simulink model "Basic_DMT"  (R2014b)
settings: Solver=FixedStepDiscrete  SolverMode=SingleTasking  StartTime=0.0  StopTime=25e-6-14e-9*24  RelTol=1e-3
PreLoadFcn:
  | userName = getenv('UserName');
  | 
  | if strcmp(userName,'Tim')
  | cd C:\Users\Tim\Documents\GitHub\MA_1\Basic_DMT
  | else
  | cd C:\Users\Tim-UML\Documents\GitHub\MA_1\Basic_DMT
  | end
InitFcn:
  | userName = getenv('UserName');
  | 
  | if strcmp(userName,'Tim')
  | cd C:\Users\Tim\Documents\GitHub\MA_1\Basic_DMT
  | else
  | cd C:\Users\Tim-UML\Documents\GitHub\MA_1\Basic_DMT
  | end
values from neighbouring files (symbols this model uses):
  a0 = 0.21194908595403703    (= 0.211949085954)    [initScript.m]
  a1 = 0.576101828091926    (= 0.576101828092)    [initScript.m]
  a2 = a0    (= 0.211949085954)    [initScript.m]
  beta = 1    [initScript.m]
  bitPerSymb = 4    [initScript.m]
  chanDownFact = Tchan/SystemPeriod    [initScript.m]
  fftLen = 16    [initScript.m]
  fftLenActive = fftLenDMT    (= 32)    [initScript.m]
  fftLenDMT = 2*fftLen    (= 32)    [initScript.m]
  GI_Active = GI_LenDMT    (= 0)    [initScript.m]
  GI_Len = 0    [initScript.m]
  GI_LenDMT = 0    [initScript.m]
  M = log2(fftLen)    [initScript.m]
  sysgenSystemPeriod = 4e-9    (= 4e-09)    [initScript.m]
  SystemPeriod = 4e-9    (= 4e-09)    [initScript.m]
  upsampleFactor = 1    [initScript.m]
  usedSubCar = 14    [initScript.m]
undefined symbols (not defined in the file or in its folder): bitCount, get, modu_mode, Tb, Ts
libraries: xbsIndex_r4 x822, commdigbbndam3 x59, simulink x42, dspsigops x7, commrandsrc2 x6, dspbuff3 x4, dspxfrm3 x3, dspswit3 x2, commseqgen2 x1, dsparch4 x1, commutil2 x1, dspsnks4 x1
(part 2 of 10)

== system Basic_DMT/OFDMorDMT ==
  note: 1) Add Subsystem or Model blocks as valid variant choices.
      | 2) You cannot connect blocks at this level. At simulation, connectivity is automatically
      | determined, based on the active variant and port name matching.
  In1 : Inport
  DMT : Subsystem  VariantControl=dmtOfdm==2
  OFDM : Subsystem  VariantControl=dmtOfdm==1
  Out1 : Outport

== system Basic_DMT/PIS  ==
  Sub1 : Inport
  Sub2 : Inport  Port=2
  Sub3 : Inport  Port=3
  Sub4 : Inport  Port=4
  Sub5 : Inport  Port=5
  Sub6 : Inport  Port=6
  Sub7 : Inport  Port=7
  Sub8 : Inport  Port=8
  Sub9 : Inport  Port=9
  Sub10 : Inport  Port=10
  Sub11 : Inport  Port=11
  Sub12 : Inport  Port=12
  Sub13 : Inport  Port=13
  Sub14 : Inport  Port=14
  sg_Bit : Inport  Port=15
  Add3 : Sum  Inputs=+-
  Delay : Delay  DelayLength=1  InitialCondition=0
  Gateway Out : xbsIndex_r4/Gateway Out  inherit_from_input=on  hdl_port=off  rows=1  columns=1  UseAsDAC=off  DACChannel='1'  interface=None  automatic_assignment=on  address_offset=hex2dec('00')  intf_description=''  timing_constraint=None  locs_specified=off  LOCs={}  io_standard={}  block_type=gatewayout
  Mux : Mux  Inputs=14
  Scope5 : Scope  Commented=on  NumInputPorts=3
      settings: YMin=-5~-5~-5  YMax=5~5~5  SaveName=ScopeData29
  Unbuffer : Unbuffer  SampleBasedProcessing=Same as frame based
  Out : Outport
  wires:
  Mux/1 -> Unbuffer/1
  Sub2/1 -> Mux/2
  Sub1/1 -> Mux/1
  Gateway Out/1 -> Scope5/2, Add3/2
  Add3/1 -> Scope5/3
  Unbuffer/1 -> Delay/1
  Delay/1 -> Add3/1, Scope5/1, Out/1
  sg_Bit/1 -> Gateway Out/1
  Sub4/1 -> Mux/4
  Sub3/1 -> Mux/3
  Sub6/1 -> Mux/6
  Sub5/1 -> Mux/5
  Sub8/1 -> Mux/8
  Sub7/1 -> Mux/7
  Sub10/1 -> Mux/10
  Sub9/1 -> Mux/9
  Sub11/1 -> Mux/11
  Sub13/1 -> Mux/13
  Sub14/1 -> Mux/14
  Sub12/1 -> Mux/12

== system Basic_DMT/Receiver ==

== system Basic_DMT/SIP  ==
  S1 : Inport
  Debug1 : Inport  Port=2
  Debug2 : Inport  Port=3
  Add1 : Sum  Inputs=+-
  Assert DIfferent Output : Subsystem
  Buffer : Buffer  N=usedSubCar*bitPerSymb  TreatMby1Signals=One channel
  Constant1 : Constant  Value=0  SampleTime=SystemPeriod
  Data Store Memory : DataStoreMemory  DataStoreName=state  OutDataTypeStr=double
  Data Store Memory1 : DataStoreMemory  DataStoreName=k  OutDataTypeStr=double
  Data Store Memory2 : DataStoreMemory  DataStoreName=loopCount  OutDataTypeStr=double
  Data Store Memory3 : DataStoreMemory  DataStoreName=subCar  InitialValue=1  OutDataTypeStr=double
  Delay : Delay  DelayLength=1  InitialCondition=0
  Delay1 : Delay  DelayLength=65  InitialCondition=0
  Delay2 : Delay  DelayLength=1  InitialCondition=0
  Demux : Demux  Outputs=14
  Index Vector : MultiPortSwitch  DataPortOrder=Zero-based contiguous  Inputs=2  zeroidx=on
  MATLAB Function : MATLAB Function  TreatAsAtomicUnit=on  SystemSampleTime=SystemPeriod
  Queue : dspbuff3/Queue  depth=64  trigger=Non-zero sample  overflow=Dynamic reallocation  pes=Warning  eso=off  fso=off  nso=on  clr=off  clrOutport=off  adf=off
  Scope1 : Scope  NumInputPorts=3
      settings: YMin=0~0~0  YMax=1~1~1  SaveName=ScopeData70
  Scope2 : Scope  NumInputPorts=2
      settings: YMin=0~-0  YMax=1~2  SaveName=ScopeData71
  Scope3 : Scope  NumInputPorts=3
      settings: YMin=0~0~-1  YMax=1~1~1  SaveName=ScopeData73
  Zero-Order Hold : ZeroOrderHold  SampleTime=SystemPeriod
  Zero-Order Hold1 : ZeroOrderHold  SampleTime=Ts
  Sub1 : Outport
  Sub2 : Outport  Port=2
  Sub3 : Outport  Port=3
  Sub4 : Outport  Port=4
  Sub5 : Outport  Port=5
  Sub6 : Outport  Port=6
  Sub7 : Outport  Port=7
  Sub8 : Outport  Port=8
  Sub9 : Outport  Port=9
  Sub10 : Outport  Port=10
  Sub11 : Outport  Port=11
  Sub12 : Outport  Port=12
  Sub13 : Outport  Port=13
  Sub14 : Outport  Port=14
  wires:
  Demux/2 -> Assert DIfferent Output/2(In2), Sub2/1
  Buffer/1 -> Demux/1
  Demux/1 -> Assert DIfferent Output/1(In1), Sub1/1
  Debug1/1 -> Assert DIfferent Output/3(In3)
  Debug2/1 -> Assert DIfferent Output/4(In4)
  Zero-Order Hold/1 -> Zero-Order Hold1/1, Scope2/1, Queue/1
  Demux/3 -> Sub3/1
  Demux/4 -> Sub4/1
  Demux/5 -> Sub5/1
  Demux/6 -> Sub6/1
  Demux/7 -> Sub7/1
  Demux/8 -> Sub8/1
  Demux/9 -> Sub9/1
  Demux/10 -> Sub10/1
  Demux/11 -> Sub11/1
  Demux/14 -> Sub14/1
  Demux/13 -> Sub13/1
  Demux/12 -> Sub12/1
  Queue/1 -> Index Vector/3
  Constant1/1 -> Index Vector/2
  Queue/2 -> Delay/1
  MATLAB Function/1(sel) -> Index Vector/1, Scope1/1
  Delay/1 -> MATLAB Function/1(num), Scope2/2
  Index Vector/1 -> Delay2/1
  Zero-Order Hold1/1 -> Delay1/1
  Add1/1 -> Scope3/3
  Delay1/1 -> Add1/2, Scope3/2
  MATLAB Function/2(push) -> Scope1/2, Queue/2
  MATLAB Function/3(pop) -> Scope1/3, Queue/3
  S1/1 -> Zero-Order Hold/1
  Delay2/1 -> Buffer/1, Scope3/1, Add1/1

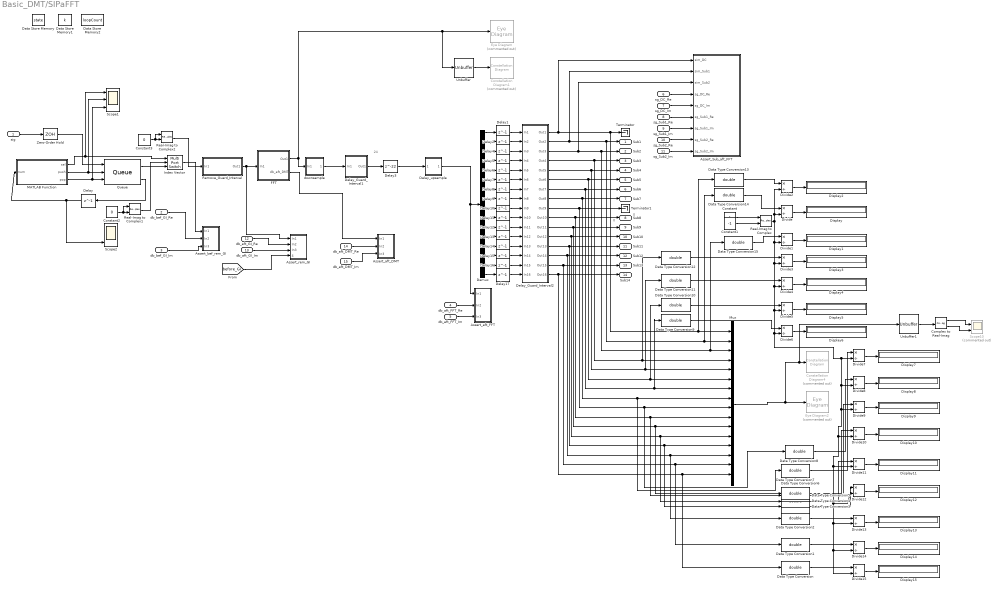
== system Basic_DMT/SIPaFFT ==
  note: 24
  note: 0
  note: 0
  sig : Inport
  db_bef_GI_Re : Inport  Port=2
  db_bef_GI_Im : Inport  Port=3
  db_aft_FFT_Re : Inport  Port=4
  db_aft_FFT_Im : Inport  Port=5
  sg_DC_Re : Inport  Port=6
  sg_DC_Im : Inport  Port=7
  sg_Sub1_Re : Inport  Port=8
  sg_Sub1_Im : Inport  Port=9
  sg_Sub2_Re : Inport  Port=10
  sg_Sub2_Im : Inport  Port=11
  db_aft_GI_Re : Inport  Port=12
  db_aft_GI_Im : Inport  Port=13
  db_aft_DMT_Re : Inport  Port=14
  db_aft_DMT_Im : Inport  Port=15
  Assert_Sub_aft_FFT : Subsystem
  Assert_aft_DMT : Subsystem
  Assert_aft_FFT : Subsystem
  Assert_bef_rem_GI : Subsystem
  Assert_rem_GI : Subsystem
  Complex to Real-Imag : ComplexToRealImag
  Constant : Constant
  Constant1 : Constant  Value=-1
  Constant2 : Constant  Value=0  SampleTime=SystemPeriod
  Constant3 : Constant  Value=0  SampleTime=SystemPeriod
  Constellation Diagram1 : ConstellationDiagram  Commented=on
  Constellation Diagram4 : ConstellationDiagram  Commented=on
  Data Store Memory : DataStoreMemory  DataStoreName=state  OutDataTypeStr=double
  Data Store Memory1 : DataStoreMemory  DataStoreName=k  OutDataTypeStr=double
  Data Store Memory2 : DataStoreMemory  DataStoreName=loopCount  OutDataTypeStr=double
  Data Type Conversion{,1..15} (16 alike) : DataTypeConversion  OutDataTypeStr=double
  Delay : Delay  DelayLength=1  InitialCondition=0
  Delay{1..2,4..17} (16 alike) : Delay  DelayLength=1  InitialCondition=0  InputProcessing=Columns as channels (frame based)
  Delay3 : Delay  DelayLength=22  InitialCondition=0  InputProcessing=Columns as channels (frame based)
  Delay_Guard_Interval1 : Subsystem  Variant=on
  Delay_Guard_Interval2 : Subsystem  Variant=on
  Delay_upsample : Subsystem  Variant=on
  Demux : Demux  Outputs=16
  Display{,1..15} (16 alike) : Display
  Divide{,1..15} (16 alike) : Product  Inputs=*/
  Eye Diagram : EyeDiagram  Commented=on
  Eye Diagram2 : EyeDiagram  Commented=on
  FFT : Subsystem  Variant=on
  Index Vector : MultiPortSwitch  DataPortOrder=Zero-based contiguous  Inputs=2  zeroidx=on
  MATLAB Function : MATLAB Function  TreatAsAtomicUnit=on  SystemSampleTime=SystemPeriod
  Mux : Mux  Inputs=16
  Queue : dspbuff3/Queue  depth=64  trigger=Non-zero sample  overflow=Dynamic reallocation  pes=Warning  eso=off  fso=off  nso=on  clr=off  clrOutport=off  adf=off
  Real-Imag to Complex : RealImagToComplex
  Real-Imag to Complex1 : RealImagToComplex
  Real-Imag to Complex2 : RealImagToComplex
  Remove_Guard_Interval : Subsystem  Variant=on
  Scope1 : Scope  NumInputPorts=3
      settings: YMin=0~0~0  YMax=1~1~1  SaveName=ScopeData75
  Scope10 : Scope  Commented=on  NumInputPorts=2
      settings: YMin=-5~-5  YMax=5~5  SaveName=ScopeData66
  Scope2 : Scope  NumInputPorts=3
      settings: YMin=0~0~0  YMax=1~1~1  SaveName=ScopeData76
  Terminator : Terminator
  Terminator1 : Terminator
  Unbuffer : Unbuffer  SampleBasedProcessing=Same as frame based
  Unbuffer1 : Unbuffer  SampleBasedProcessing=Same as frame based
  Zero-Order Hold : ZeroOrderHold  SampleTime=SystemPeriod
  downsample : Subsystem  Variant=on
  Sub1 : Outport
  Sub2 : Outport  Port=2
  Sub3 : Outport  Port=3
  Sub4 : Outport  Port=4
  Sub5 : Outport  Port=5
  Sub6 : Outport  Port=6
  Sub7 : Outport  Port=7
  Sub8 : Outport  Port=8
  Sub9 : Outport  Port=9
  Sub10 : Outport  Port=10
  Sub11 : Outport  Port=11
  Sub12 : Outport  Port=12
  Sub13 : Outport  Port=13
  Sub14 : Outport  Port=14
  wires:
  Demux/2 -> Delay2/1
  Demux/3 -> Delay4/1
  Demux/1 -> Delay1/1
  Demux/4 -> Delay5/1
  Demux/6 -> Delay7/1
  Demux/5 -> Delay6/1
  Demux/7 -> Delay8/1
  Demux/8 -> Delay9/1
  db_bef_GI_Im/1 -> Assert_bef_rem_GI/3(In3)
  db_bef_GI_Re/1 -> Assert_bef_rem_GI/2(In2)
  db_aft_FFT_Re/1 -> Assert_aft_FFT/2(In2)
  db_aft_FFT_Im/1 -> Assert_aft_FFT/3(In3)
  sg_DC_Re/1 -> Assert_Sub_aft_FFT/4(sg_DC_Re)
  sg_DC_Im/1 -> Assert_Sub_aft_FFT/5(sg_DC_Im)
  sg_Sub1_Re/1 -> Assert_Sub_aft_FFT/6(sg_Sub1_Re)
  sg_Sub1_Im/1 -> Assert_Sub_aft_FFT/7(sg_Sub1_Im)
  sg_Sub2_Re/1 -> Assert_Sub_aft_FFT/8(sg_Sub2_Re)
  sg_Sub2_Im/1 -> Assert_Sub_aft_FFT/9(sg_Sub2_Im)
  Delay3/1 -> Delay_upsample/1(In1)
  Delay1/1 -> Delay_Guard_Interval2/1(In1)
  db_aft_GI_Im/1 -> Assert_rem_GI/3(In3)
  db_aft_GI_Re/1 -> Assert_rem_GI/2(In2)
  [before_GI] -> Assert_rem_GI/4(before_GI)
  Index Vector/1 -> Assert_bef_rem_GI/1(In1)
  Demux/16 -> Delay17/1
  Demux/15 -> Delay16/1
  Demux/14 -> Delay15/1
  Demux/13 -> Delay14/1
  Demux/12 -> Delay13/1
  Demux/11 -> Delay12/1
  Demux/10 -> Delay11/1
  Demux/9 -> Delay10/1
  Delay4/1 -> Delay_Guard_Interval2/3(In3)
  Delay5/1 -> Delay_Guard_Interval2/4(In4)
  Delay2/1 -> Delay_Guard_Interval2/2(In2)
  Delay6/1 -> Delay_Guard_Interval2/5(In5)
  Delay7/1 -> Delay_Guard_Interval2/6(In6)
  Delay8/1 -> Delay_Guard_Interval2/7(In7)
  Delay9/1 -> Delay_Guard_Interval2/8(In8)
  Delay10/1 -> Delay_Guard_Interval2/9(In9)
  Delay11/1 -> Delay_Guard_Interval2/10(In10)
  Delay12/1 -> Delay_Guard_Interval2/11(In11)
  Delay13/1 -> Delay_Guard_Interval2/12(In12)
  Delay14/1 -> Delay_Guard_Interval2/13(In13)
  Delay15/1 -> Delay_Guard_Interval2/14(In14)
  Delay16/1 -> Delay_Guard_Interval2/15(In15)
  Delay17/1 -> Delay_Guard_Interval2/16(In16)
  Delay_Guard_Interval1/1(Out1) -> Delay3/1
  Remove_Guard_Interval/1(Out1) -> FFT/1(In1), Assert_rem_GI/1(In1)
  downsample/1(Out1) -> Delay_Guard_Interval1/1(In1)
  Delay_upsample/1(Out1) -> Assert_aft_FFT/1(In1), Demux/1
  FFT/1(Out1) -> downsample/1(In1), Unbuffer/1, Eye Diagram/1
  db_aft_DMT_Im/1 -> Assert_aft_DMT/3(In3)
  db_aft_DMT_Re/1 -> Assert_aft_DMT/2(In2)
  FFT/2(db_aft_DMT) -> Assert_aft_DMT/1(In1)
  Delay_Guard_Interval2/2(Out2) -> Assert_Sub_aft_FFT/2(sim_Sub1), Data Type Conversion14/1, Mux/2, Sub1/1
  Delay_Guard_Interval2/4(Out4) -> Mux/4, Data Type Conversion12/1, Sub3/1
  Delay_Guard_Interval2/5(Out5) -> Data Type Conversion11/1, Mux/5, Sub4/1
  Delay_Guard_Interval2/6(Out6) -> Data Type Conversion10/1, Mux/6, Sub5/1
  Delay_Guard_Interval2/7(Out7) -> Data Type Conversion9/1, Mux/7, Sub6/1
  Delay_Guard_Interval2/9(Out9) -> Data Type Conversion8/1, Mux/9, Terminator1/1
  Delay_Guard_Interval2/10(Out10) -> Data Type Conversion5/1, Mux/10, Sub8/1
  Delay_Guard_Interval2/12(Out12) -> Data Type Conversion4/1, Mux/12, Sub10/1
  Delay_Guard_Interval2/15(Out15) -> Sub13/1, Data Type Conversion1/1, Mux/15
  Delay_Guard_Interval2/14(Out14) -> Sub12/1, Data Type Conversion2/1, Mux/14
  Delay_Guard_Interval2/13(Out13) -> Sub11/1, Data Type Conversion3/1, Mux/13
  Delay_Guard_Interval2/11(Out11) -> Data Type Conversion6/1, Mux/11, Sub9/1
  Mux/1 -> Unbuffer1/1, Constellation Diagram4/1, Eye Diagram2/1
  Unbuffer/1 -> Constellation Diagram1/1
  Constant/1 -> Real-Imag to Complex/1
  Divide/1 -> Display/1
  Delay_Guard_Interval2/3(Out3) -> Assert_Sub_aft_FFT/3(sim_Sub2), Mux/3, Data Type Conversion15/1, Sub2/1
  Constant1/1 -> Real-Imag to Complex/2
  Divide1/1 -> Display1/1
  Delay_Guard_Interval2/1(Out1) -> Data Type Conversion13/1, Mux/1, Terminator/1, Assert_Sub_aft_FFT/1(sim_DC)
  Real-Imag to Complex/1 -> Divide2/2, Divide/2, Divide15/2, Divide14/2, Divide13/2, Divide12/2, Divide11/2, Divide10/2, Divide9/2, Divide8/2, Divide7/2, Divide6/2, Divide5/2, Divide4/2, Divide3/2, Divide1/2
  Divide2/1 -> Display2/1
  Divide3/1 -> Display3/1
  Divide4/1 -> Display4/1
  Divide5/1 -> Display5/1
  Divide6/1 -> Display6/1
  Divide7/1 -> Display7/1
  Divide8/1 -> Display8/1
  Divide9/1 -> Display9/1
  Divide10/1 -> Display10/1
  Divide11/1 -> Display11/1
  Divide12/1 -> Display12/1
  Divide13/1 -> Display13/1
  Divide14/1 -> Display14/1
  Divide15/1 -> Display15/1
  Delay_Guard_Interval2/16(Out16) -> Data Type Conversion/1, Mux/16, Sub14/1
  Data Type Conversion/1 -> Divide15/1
  Data Type Conversion1/1 -> Divide14/1
  Data Type Conversion2/1 -> Divide13/1
  Data Type Conversion3/1 -> Divide12/1
  Data Type Conversion4/1 -> Divide11/1
  Data Type Conversion5/1 -> Divide9/1
  Data Type Conversion6/1 -> Divide10/1
  Data Type Conversion7/1 -> Divide7/1
  Data Type Conversion8/1 -> Divide8/1
  Data Type Conversion9/1 -> Divide6/1
  Data Type Conversion10/1 -> Divide5/1
  Data Type Conversion11/1 -> Divide4/1
  Data Type Conversion12/1 -> Divide3/1
  Data Type Conversion13/1 -> Divide2/1
  Data Type Conversion14/1 -> Divide/1
  Data Type Conversion15/1 -> Divide1/1
  Unbuffer1/1 -> Complex to Real-Imag/1
  Complex to Real-Imag/1 -> Scope10/1
  Complex to Real-Imag/2 -> Scope10/2
  Delay_Guard_Interval2/8(Out8) -> Data Type Conversion7/1, Mux/8, Sub7/1
  MATLAB Function/3(pop) -> Scope1/3, Queue/3
  MATLAB Function/2(push) -> Scope1/2, Queue/2
  sig/1 -> Zero-Order Hold/1
  Queue/1 -> Index Vector/3
  MATLAB Function/1(sel) -> Scope1/1, Index Vector/1
  Queue/2 -> Delay/1
  Delay/1 -> Scope2/3, MATLAB Function/1(num)
  Constant2/1 -> Real-Imag to Complex1/2, Real-Imag to Complex1/1
  Zero-Order Hold/1 -> Queue/1
  Real-Imag to Complex2/1 -> Remove_Guard_Interval/1(In1)
  Real-Imag to Complex1/1 -> Index Vector/2
  Constant3/1 -> Real-Imag to Complex2/2, Real-Imag to Complex2/1

== system Basic_DMT/Subsystem ==

== system Basic_DMT/Sysgen S//P1 ==
  " System Generator" : xbsIndex_r4/ System Generator  Tag=genX  xilinxfamily=zynq  part=xc7z020  speed=-1  package=clg400  synthesis_tool=Vivado  clock_wrapper=Clock Enables  directory=./netlist  proj_type=Vivado  Synth_file=Vivado Synthesis Defaults  Impl_file=Vivado Implementation Defaults  testbench=on  simulink_period=Ts  sysclk_period=10  dcm_input_clock_period=10  incr_netlist=off  trim_vbits=Everywhere in SubSystem  dbl_ovrd=According to Block Masks  core_generation=According to Block Masks  run_coregen=off  deprecated_control=off  eval_field=0  block_type=sysgen
  Bernoulli Binary Generator : commrandsrc2/Bernoulli Binary Generator  P=0.5  seed=1604198  Ts=Tb  frameBased=off  sampPerFrame=1  orient=off  outDataType=boolean
      settings: AttributesFormatString=|
      | Sample Time= %<Ts>
      | Prob zero=%<P>
  BitBasher : xbsIndex_r4/BitBasher  bitexpr=|  display_expr=on  sr_1=y1  arith_type1=Unsigned  bin_pt1=0  sr_2=y2  arith_type2=Unsigned  bin_pt2=0  sr_3=3  arith_type3=Unsigned  bin_pt3=0  sr_4=4  arith_type4=Unsigned  bin_pt4=0  dbl_ovrd=off  block_type=bitbasher
      | y1={a[7:4]}
      | y2={a[3:0]}
  Buffer : Buffer  N=8  TreatMby1Signals=One channel
  Check Static Range1 : simulink/Model Verification/Check  Static Range  Description=0 <= u <= 0  max=0  max_included=on  min=0  min_included=on  enabled=on  stopWhenAssertionFail=on  export=off  icon=graphic
  Check Static Range2 : simulink/Model Verification/Check  Static Range  Description=0 <= u <= 0  max=0  max_included=on  min=0  min_included=on  enabled=on  stopWhenAssertionFail=on  export=off  icon=graphic
  Clock Probe1 : xbsIndex_r4/Clock Probe  block_type=clkprobe
      settings: infoedit="Clock probe.  Produces an output of type double that mirrors the hardware system clock.<br><br>Hardware notes:  This block is ignored when hardware is generated."
  Counter Limited1 : simulink/Sources/Counter Limited  uplimit=1  tsamp=Tb
  Delay : Delay  DelayLength=1  InitialCondition=0
  Delay1 : Delay  DelayLength=1  InitialCondition=0
  Demux : Demux  Outputs=2
  Gateway In1 : xbsIndex_r4/Gateway In  gui_display_data_type=Fixed-point  arith_type=Unsigned  n_bits=1  bin_pt=0  preci_type=Single  exp_width=8  frac_width=24  rows=1  columns=1  quantization="Round  (unbiased: +/- Inf)"  overflow=Saturate  period=Ts  UseAsADC=off  ADCChannel='1'  interface=None  automatic_assignment=on  address_offset=hex2dec('00')  intf_description=''  timing_constraint=None  locs_specified=off  LOCs={}  io_standard={}  inherit_from_input=off  hdl_port=on  dbl_ovrd=off  block_type=gatewayin
  Gateway Out : xbsIndex_r4/Gateway Out  inherit_from_input=on  hdl_port=off  rows=1  columns=1  UseAsDAC=off  DACChannel='1'  interface=None  automatic_assignment=on  address_offset=hex2dec('00')  intf_description=''  timing_constraint=None  locs_specified=off  LOCs={}  io_standard={}  block_type=gatewayout
  Gateway Out1 : xbsIndex_r4/Gateway Out  inherit_from_input=on  hdl_port=off  rows=1  columns=1  UseAsDAC=off  DACChannel='1'  interface=None  automatic_assignment=on  address_offset=hex2dec('00')  intf_description=''  timing_constraint=None  locs_specified=off  LOCs={}  io_standard={}  block_type=gatewayout
  Manual Switch : ManualSwitch  CurrentSetting=0
  Parallel to Serial : xbsIndex_r4/Parallel to Serial  output_order=Most Significant Word First  arith_type=Unsigned  output_bits=1  bin_pt=0  rst=off  en=off  latency=1  dbl_ovrd=off  block_type=p2s
      settings: infoedit=Each sample presented at the input becomes several samples presented serially at the output.
  Parallel to Serial1 : xbsIndex_r4/Parallel to Serial  output_order=Most Significant Word First  arith_type=Unsigned  output_bits=1  bin_pt=0  rst=off  en=off  latency=1  dbl_ovrd=off  block_type=p2s
      settings: infoedit=Each sample presented at the input becomes several samples presented serially at the output.
  Scope : Scope  NumInputPorts=8
      settings: YMin=-5~-5~-5~-5~-5~-5~-5~-5  YMax=5~5~5~5~5~5~5~5  SaveName=ScopeData4
  Serial to Parallel : xbsIndex_r4/Serial to Parallel  input_order=Most Significant Word First  arith_type=Unsigned  output_bits=8  bin_pt=0  rst=off  en=off  latency=1  dbl_ovrd=off  block_type=s2p
      settings: infoedit=Groups of samples presented serially at the input become single samples presented at the output.
  Subtract : Sum  Inputs=+-
  Subtract1 : Sum  Inputs=+-
  Unbuffer : Unbuffer  SampleBasedProcessing=Same as frame based
  Unbuffer1 : Unbuffer  SampleBasedProcessing=Same as frame based
  wires:
  Gateway In1/1 -> Serial to Parallel/1
  BitBasher/1 -> Parallel to Serial/1
  BitBasher/2 -> Parallel to Serial1/1
  Bernoulli Binary Generator/1 -> Manual Switch/2
  Counter Limited1/1 -> Manual Switch/1
  Demux/2 -> Unbuffer/1
  Buffer/1 -> Demux/1
  Demux/1 -> Unbuffer1/1
  Manual Switch/1 -> Scope/8, Buffer/1, Gateway In1/1
  Gateway Out/1 -> Scope/3, Subtract/2
  Unbuffer/1 -> Delay1/1
  Unbuffer1/1 -> Delay/1
  Serial to Parallel/1 -> BitBasher/1
  Parallel to Serial/1 -> Gateway Out/1
  Parallel to Serial1/1 -> Gateway Out1/1
  Delay/1 -> Scope/1, Subtract/1
  Subtract/1 -> Check Static Range1/1, Scope/5
  Gateway Out1/1 -> Scope/4, Subtract1/2
  Delay1/1 -> Scope/2, Subtract1/1
  Clock Probe1/1 -> Scope/7
  Subtract1/1 -> Check Static Range2/1, Scope/6

== system Basic_DMT/Sysgen_AWGN ==
  note: 1) Add Subsystem or Model blocks as valid variant choices.
      | 2) You cannot connect blocks at this level. At simulation, connectivity is automatically
      | determined, based on the active variant and port name matching.
  Re : Inport
  Im : Inport  Port=2
  No_AWGN : Subsystem  VariantControl=AWGN==1
  Yes_AWGN : Subsystem  VariantControl=AWGN==2
  Re_out : Outport
  Im_out : Outport  Port=2
  db_bool : Outport  Port=3
  db_full : Outport  Port=4

== system Basic_DMT/Sysgen_Channel ==
  note: 1) Add Subsystem or Model blocks as valid variant choices.
      | 2) You cannot connect blocks at this level. At simulation, connectivity is automatically
      | determined, based on the active variant and port name matching.
  Re : Inport
  Im : Inport  Port=2
  No_channel : Subsystem  VariantControl=channel==1
  Yes_Channel : Subsystem  VariantControl=channel==2
  Re_out : Outport
  Im_out : Outport  Port=2

== system Basic_DMT/Sysgen_Demodulation ==
  Re_Sub1 : Inport
  Im_Sub1 : Inport  Port=2
  Re_Sub2 : Inport  Port=3
  Im_Sub2 : Inport  Port=4
  Re_Sub3 : Inport  Port=5
  Im_Sub3 : Inport  Port=6
  Re_Sub4 : Inport  Port=7
  Im_Sub4 : Inport  Port=8
  Re_Sub5 : Inport  Port=9
  Im_Sub5 : Inport  Port=10
  Re_Sub6 : Inport  Port=11
  Im_Sub6 : Inport  Port=12
  Re_Sub7 : Inport  Port=13
  Im_Sub7 : Inport  Port=14
  Re_Sub8 : Inport  Port=15
  Im_Sub8 : Inport  Port=16
  Re_Sub9 : Inport  Port=17
  Im_Sub9 : Inport  Port=18
  Re_Sub10 : Inport  Port=19
  Im_Sub10 : Inport  Port=20
  Re_Sub11 : Inport  Port=21
  Im_Sub11 : Inport  Port=22
  Re_Sub12 : Inport  Port=23
  Im_Sub12 : Inport  Port=24
  Re_Sub13 : Inport  Port=25
  Im_Sub13 : Inport  Port=26
  Re_Sub14 : Inport  Port=27
  Im_Sub14 : Inport  Port=28
  MCode{1..14} (14 alike) : xbsIndex_r4/MCode  mfname=Demod_16QAM  explicit_period=off  period=1  inputsTable={'boundInpExpr'=>['',''],'inputs'=>['I','Q']}  outputsTable={'outputs'=>['y1'],'suppressOut'=>['off']}  enable_stdout=off  enable_debug=off  suppress_output=on  defparams={}  hide_port_list={}  dbl_ovrd=off  block_type=mcode
  Bit_Sub1 : Outport
  Bit_Sub2 : Outport  Port=2
  Bit_Sub3 : Outport  Port=3
  Bit_Sub4 : Outport  Port=4
  Bit_Sub5 : Outport  Port=5
  Bit_Sub6 : Outport  Port=6
  Bit_Sub7 : Outport  Port=7
  Bit_Sub8 : Outport  Port=8
  Bit_Sub9 : Outport  Port=9
  Bit_Sub10 : Outport  Port=10
  Bit_Sub11 : Outport  Port=11
  Bit_Sub12 : Outport  Port=12
  Bit_Sub13 : Outport  Port=13
  Bit_Sub14 : Outport  Port=14
  wires:
  Re_Sub1/1 -> MCode1/1
  Im_Sub1/1 -> MCode1/2
  Re_Sub2/1 -> MCode2/1
  Im_Sub2/1 -> MCode2/2
  MCode1/1 -> Bit_Sub1/1
  MCode2/1 -> Bit_Sub2/1
  Re_Sub3/1 -> MCode3/1
  Im_Sub3/1 -> MCode3/2
  Re_Sub4/1 -> MCode4/1
  Im_Sub4/1 -> MCode4/2
  MCode3/1 -> Bit_Sub3/1
  MCode4/1 -> Bit_Sub4/1
  Re_Sub5/1 -> MCode5/1
  Im_Sub5/1 -> MCode5/2
  Re_Sub6/1 -> MCode6/1
  Im_Sub6/1 -> MCode6/2
  MCode5/1 -> Bit_Sub5/1
  MCode6/1 -> Bit_Sub6/1
  Re_Sub7/1 -> MCode7/1
  Im_Sub7/1 -> MCode7/2
  Re_Sub8/1 -> MCode8/1
  Im_Sub8/1 -> MCode8/2
  MCode7/1 -> Bit_Sub7/1
  MCode8/1 -> Bit_Sub8/1
  Re_Sub9/1 -> MCode9/1
  Im_Sub9/1 -> MCode9/2
  Re_Sub10/1 -> MCode10/1
  Im_Sub10/1 -> MCode10/2
  MCode9/1 -> Bit_Sub9/1
  MCode10/1 -> Bit_Sub10/1
  Re_Sub11/1 -> MCode11/1
  Im_Sub11/1 -> MCode11/2
  Re_Sub12/1 -> MCode12/1
  Im_Sub12/1 -> MCode12/2
  MCode11/1 -> Bit_Sub11/1
  MCode12/1 -> Bit_Sub12/1
  Re_Sub13/1 -> MCode13/1
  Im_Sub13/1 -> MCode13/2
  Re_Sub14/1 -> MCode14/1
  Im_Sub14/1 -> MCode14/2
  MCode13/1 -> Bit_Sub13/1
  MCode14/1 -> Bit_Sub14/1

== system Basic_DMT/Sysgen_IFFTaPIS ==
  Re_Sub1 : Inport
  Im_Sub1 : Inport  Port=2
  Re_Sub2 : Inport  Port=3
  Im_Sub2 : Inport  Port=4
  Re_Sub3 : Inport  Port=5
  Im_Sub3 : Inport  Port=6
  Re_Sub4 : Inport  Port=7
  Im_Sub4 : Inport  Port=8
  Re_Sub5 : Inport  Port=9
  Im_Sub5 : Inport  Port=10
  Re_Sub6 : Inport  Port=11
  Im_Sub6 : Inport  Port=12
  Re_Sub7 : Inport  Port=13
  Im_Sub7 : Inport  Port=14
  Re_Sub8 : Inport  Port=15
  Im_Sub8 : Inport  Port=16
  Re_Sub9 : Inport  Port=17
  Im_Sub9 : Inport  Port=18
  Re_Sub10 : Inport  Port=19
  Im_Sub10 : Inport  Port=20
  Re_Sub11 : Inport  Port=21
  Im_Sub11 : Inport  Port=22
  Re_Sub12 : Inport  Port=23
  Im_Sub12 : Inport  Port=24
  Re_Sub13 : Inport  Port=25
  Im_Sub13 : Inport  Port=26
  Re_Sub14 : Inport  Port=27
  Im_Sub14 : Inport  Port=28
  Guard_Interval : Subsystem  Variant=on
  OFDMorDMT : Subsystem  Variant=on
  Re : Outport
  Im : Outport  Port=2
  Db_aft_frame_Re : Outport  Port=3
  Db_aft_frame_Im : Outport  Port=4
  Db_aft_FFT_Re : Outport  Port=5
  Db_aft_FFT_Im : Outport  Port=6
  wires:
  Re_Sub1/1 -> OFDMorDMT/1(Re_Sub1)
  Im_Sub2/1 -> OFDMorDMT/4(Im_Sub2)
  OFDMorDMT/4(Debug_Im) -> Db_aft_frame_Im/1
  OFDMorDMT/3(Debug_Re) -> Db_aft_frame_Re/1
  Re_Sub2/1 -> OFDMorDMT/3(Re_Sub2)
  Im_Sub1/1 -> OFDMorDMT/2(Im_Sub1)
  Guard_Interval/1(Re) -> Re/1
  Guard_Interval/2(Im) -> Im/1
  OFDMorDMT/2(Im) -> Db_aft_FFT_Im/1, Guard_Interval/2(Im_In)
  OFDMorDMT/1(Re) -> Db_aft_FFT_Re/1, Guard_Interval/1(Re_In)
  Re_Sub3/1 -> OFDMorDMT/5(Re_Sub3)
  Im_Sub3/1 -> OFDMorDMT/6(Im_Sub3)
  Re_Sub4/1 -> OFDMorDMT/7(Re_Sub4)
  Im_Sub4/1 -> OFDMorDMT/8(Im_Sub4)
  Im_Sub5/1 -> OFDMorDMT/10(Im_Sub5)
  Re_Sub6/1 -> OFDMorDMT/11(Re_Sub6)
  Im_Sub6/1 -> OFDMorDMT/12(Im_Sub6)
  Re_Sub7/1 -> OFDMorDMT/13(Re_Sub7)
  Im_Sub7/1 -> OFDMorDMT/14(Im_Sub7)
  Re_Sub8/1 -> OFDMorDMT/15(Re_Sub8)
  Im_Sub8/1 -> OFDMorDMT/16(Im_Sub8)
  Re_Sub9/1 -> OFDMorDMT/17(Re_Sub9)
  Im_Sub9/1 -> OFDMorDMT/18(Im_Sub9)
  Re_Sub10/1 -> OFDMorDMT/19(Re_Sub10)
  Im_Sub10/1 -> OFDMorDMT/20(Im_Sub10)
  Re_Sub11/1 -> OFDMorDMT/21(Re_Sub11)
  Im_Sub11/1 -> OFDMorDMT/22(Im_Sub11)
  Re_Sub12/1 -> OFDMorDMT/23(Re_Sub12)
  Im_Sub12/1 -> OFDMorDMT/24(Im_Sub12)
  Re_Sub13/1 -> OFDMorDMT/25(Re_Sub13)
  Im_Sub13/1 -> OFDMorDMT/26(Im_Sub13)
  Re_Sub14/1 -> OFDMorDMT/27(Re_Sub14)
  Im_Sub14/1 -> OFDMorDMT/28(Im_Sub14)
  Re_Sub5/1 -> OFDMorDMT/9(Re_Sub5)

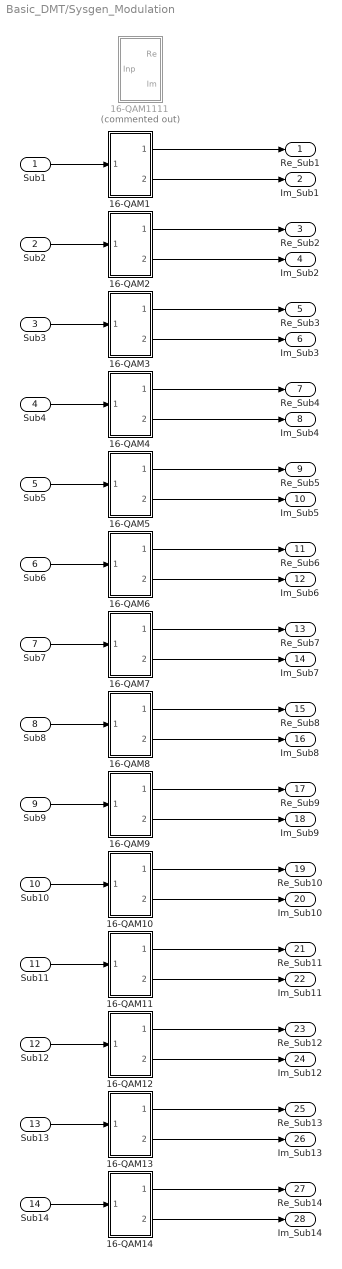
== system Basic_DMT/Sysgen_Modulation ==
  Sub1 : Inport
  Sub2 : Inport  Port=2
  Sub3 : Inport  Port=3
  Sub4 : Inport  Port=4
  Sub5 : Inport  Port=5
  Sub6 : Inport  Port=6
  Sub7 : Inport  Port=7
  Sub8 : Inport  Port=8
  Sub9 : Inport  Port=9
  Sub10 : Inport  Port=10
  Sub11 : Inport  Port=11
  Sub12 : Inport  Port=12
  Sub13 : Inport  Port=13
  Sub14 : Inport  Port=14
  16-QAM1 : Subsystem
  16-QAM10 : Subsystem
  16-QAM11 : Subsystem
  16-QAM1111 : Subsystem  Commented=on
  16-QAM12 : Subsystem
  16-QAM13 : Subsystem
  16-QAM14 : Subsystem
  16-QAM2 : Subsystem
  16-QAM3 : Subsystem
  16-QAM4 : Subsystem
  16-QAM5 : Subsystem
  16-QAM6 : Subsystem
  16-QAM7 : Subsystem
  16-QAM8 : Subsystem
  16-QAM9 : Subsystem
  Re_Sub1 : Outport
  Im_Sub1 : Outport  Port=2
  Re_Sub2 : Outport  Port=3
  Im_Sub2 : Outport  Port=4
  Re_Sub3 : Outport  Port=5
  Im_Sub3 : Outport  Port=6
  Re_Sub4 : Outport  Port=7
  Im_Sub4 : Outport  Port=8
  Re_Sub5 : Outport  Port=9
  Im_Sub5 : Outport  Port=10
  Re_Sub6 : Outport  Port=11
  Im_Sub6 : Outport  Port=12
  Re_Sub7 : Outport  Port=13
  Im_Sub7 : Outport  Port=14
  Re_Sub8 : Outport  Port=15
  Im_Sub8 : Outport  Port=16
  Re_Sub9 : Outport  Port=17
  Im_Sub9 : Outport  Port=18
  Re_Sub10 : Outport  Port=19
  Im_Sub10 : Outport  Port=20
  Re_Sub11 : Outport  Port=21
  Im_Sub11 : Outport  Port=22
  Re_Sub12 : Outport  Port=23
  Im_Sub12 : Outport  Port=24
  Re_Sub13 : Outport  Port=25
  Im_Sub13 : Outport  Port=26
  Re_Sub14 : Outport  Port=27
  Im_Sub14 : Outport  Port=28
  wires:
  Sub1/1 -> 16-QAM1/1(In1)
  16-QAM1/2(Out3) -> Im_Sub1/1
  16-QAM1/1(Out2) -> Re_Sub1/1
  Sub2/1 -> 16-QAM2/1(In1)
  16-QAM2/2(Out3) -> Im_Sub2/1
  16-QAM2/1(Out2) -> Re_Sub2/1
  Sub3/1 -> 16-QAM3/1(In1)
  16-QAM3/2(Out3) -> Im_Sub3/1
  16-QAM3/1(Out2) -> Re_Sub3/1
  Sub4/1 -> 16-QAM4/1(In1)
  16-QAM4/2(Out3) -> Im_Sub4/1
  16-QAM4/1(Out2) -> Re_Sub4/1
  Sub5/1 -> 16-QAM5/1(In1)
  16-QAM5/2(Out3) -> Im_Sub5/1
  16-QAM5/1(Out2) -> Re_Sub5/1
  Sub6/1 -> 16-QAM6/1(In1)
  16-QAM6/2(Out3) -> Im_Sub6/1
  16-QAM6/1(Out2) -> Re_Sub6/1
  Sub7/1 -> 16-QAM7/1(In1)
  16-QAM7/2(Out3) -> Im_Sub7/1
  16-QAM7/1(Out2) -> Re_Sub7/1
  Sub8/1 -> 16-QAM8/1(In1)
  16-QAM8/2(Out3) -> Im_Sub8/1
  16-QAM8/1(Out2) -> Re_Sub8/1
  Sub9/1 -> 16-QAM9/1(In1)
  16-QAM9/2(Out3) -> Im_Sub9/1
  16-QAM9/1(Out2) -> Re_Sub9/1
  Sub10/1 -> 16-QAM10/1(In1)
  16-QAM10/2(Out3) -> Im_Sub10/1
  16-QAM10/1(Out2) -> Re_Sub10/1
  Sub11/1 -> 16-QAM11/1(In1)
  16-QAM11/2(Out3) -> Im_Sub11/1
  16-QAM11/1(Out2) -> Re_Sub11/1
  Sub12/1 -> 16-QAM12/1(In1)
  16-QAM12/2(Out3) -> Im_Sub12/1
  16-QAM12/1(Out2) -> Re_Sub12/1
  Sub13/1 -> 16-QAM13/1(In1)
  16-QAM13/2(Out3) -> Im_Sub13/1
  16-QAM13/1(Out2) -> Re_Sub13/1
  Sub14/1 -> 16-QAM14/1(In1)
  16-QAM14/2(Out3) -> Im_Sub14/1
  16-QAM14/1(Out2) -> Re_Sub14/1

== system Basic_DMT/Sysgen_PIS ==
  Bit_Sub1 : Inport
  Bit_Sub2 : Inport  Port=2
  Bit_Sub3 : Inport  Port=3
  Bit_Sub4 : Inport  Port=4
  Bit_Sub5 : Inport  Port=5
  Bit_Sub6 : Inport  Port=6
  Bit_Sub7 : Inport  Port=7
  Bit_Sub8 : Inport  Port=8
  Bit_Sub9 : Inport  Port=9
  Bit_Sub10 : Inport  Port=10
  Bit_Sub11 : Inport  Port=11
  Bit_Sub12 : Inport  Port=12
  Bit_Sub13 : Inport  Port=13
  Bit_Sub14 : Inport  Port=14
  Concat : xbsIndex_r4/Concat  num_inputs=14  dbl_ovrd=off  block_type=concat
  Parallel to Serial : xbsIndex_r4/Parallel to Serial  output_order=Most Significant Word First  arith_type=Unsigned  output_bits=1  bin_pt=0  rst=off  en=off  latency=1  dbl_ovrd=off  block_type=p2s
      settings: infoedit=Each sample presented at the input becomes several samples presented serially at the output.
  Slice{1..7,13,17..21,24} (14 alike) : xbsIndex_r4/Slice  nbits=4  boolean_output=off  mode=Lower Bit Location + Width  bit1=0  base1=MSB of Input  bit0=0  base0=LSB of Input  dbl_ovrd=off  block_type=slice
  Bit : Outport
  wires:
  Slice7/1 -> Concat/1
  Bit_Sub1/1 -> Slice7/1
  Concat/1 -> Parallel to Serial/1
  Parallel to Serial/1 -> Bit/1
  Bit_Sub2/1 -> Slice1/1
  Slice1/1 -> Concat/2
  Slice3/1 -> Concat/3
  Bit_Sub3/1 -> Slice3/1
  Bit_Sub4/1 -> Slice2/1
  Slice2/1 -> Concat/4
  Slice13/1 -> Concat/5
  Bit_Sub5/1 -> Slice13/1
  Bit_Sub6/1 -> Slice4/1
  Slice4/1 -> Concat/6
  Slice6/1 -> Concat/7
  Bit_Sub7/1 -> Slice6/1
  Bit_Sub8/1 -> Slice5/1
  Slice5/1 -> Concat/8
  Slice20/1 -> Concat/9
  Bit_Sub9/1 -> Slice20/1
  Bit_Sub10/1 -> Slice17/1
  Slice17/1 -> Concat/10
  Slice19/1 -> Concat/11
  Bit_Sub11/1 -> Slice19/1
  Bit_Sub12/1 -> Slice18/1
  Slice18/1 -> Concat/12
  Slice24/1 -> Concat/13
  Bit_Sub13/1 -> Slice24/1
  Bit_Sub14/1 -> Slice21/1
  Slice21/1 -> Concat/14

== system Basic_DMT/Sysgen_SIP ==
  note: delay weg?
  Inp : Inport
  Gateway In1 : xbsIndex_r4/Gateway In  gui_display_data_type=Fixed-point  arith_type=Unsigned  n_bits=1  bin_pt=0  preci_type=Single  exp_width=8  frac_width=24  rows=1  columns=1  quantization="Round  (unbiased: +/- Inf)"  overflow=Saturate  period=Ts  UseAsADC=off  ADCChannel='1'  interface=None  automatic_assignment=on  address_offset=hex2dec('00')  intf_description=''  timing_constraint=None  locs_specified=off  LOCs={}  io_standard={}  inherit_from_input=off  hdl_port=on  dbl_ovrd=off  block_type=gatewayin
  Serial to Parallel : xbsIndex_r4/Serial to Parallel  input_order=Most Significant Word First  arith_type=Unsigned  output_bits=bitPerSymb*usedSubCar  bin_pt=0  rst=off  en=off  latency=1  dbl_ovrd=off  block_type=s2p
      settings: infoedit=Groups of samples presented serially at the input become single samples presented at the output.
  Slice1 : xbsIndex_r4/Slice  nbits=bitPerSymb  boolean_output=off  mode=Lower Bit Location + Width  bit1=0  base1=MSB of Input  bit0=7*bitPerSymb  base0=LSB of Input  dbl_ovrd=off  block_type=slice
  Slice10 : xbsIndex_r4/Slice  nbits=bitPerSymb  boolean_output=off  mode=Lower Bit Location + Width  bit1=0  base1=MSB of Input  bit0=2*bitPerSymb  base0=LSB of Input  dbl_ovrd=off  block_type=slice
  Slice11 : xbsIndex_r4/Slice  nbits=bitPerSymb  boolean_output=off  mode=Lower Bit Location + Width  bit1=0  base1=MSB of Input  bit0=3*bitPerSymb  base0=LSB of Input  dbl_ovrd=off  block_type=slice
  Slice12 : xbsIndex_r4/Slice  nbits=bitPerSymb  boolean_output=off  mode=Lower Bit Location + Width  bit1=0  base1=MSB of Input  bit0=4*bitPerSymb  base0=LSB of Input  dbl_ovrd=off  block_type=slice
  Slice13 : xbsIndex_r4/Slice  nbits=bitPerSymb  boolean_output=off  mode=Lower Bit Location + Width  bit1=0  base1=MSB of Input  bit0=6*bitPerSymb  base0=LSB of Input  dbl_ovrd=off  block_type=slice
  Slice14 : xbsIndex_r4/Slice  nbits=bitPerSymb  boolean_output=off  mode=Lower Bit Location + Width  bit1=0  base1=MSB of Input  bit0=5*bitPerSymb  base0=LSB of Input  dbl_ovrd=off  block_type=slice
  Slice2 : xbsIndex_r4/Slice  nbits=bitPerSymb  boolean_output=off  mode=Lower Bit Location + Width  bit1=0  base1=MSB of Input  bit0=8*bitPerSymb  base0=LSB of Input  dbl_ovrd=off  block_type=slice
  Slice3 : xbsIndex_r4/Slice  nbits=bitPerSymb  boolean_output=off  mode=Lower Bit Location + Width  bit1=0  base1=MSB of Input  bit0=9*bitPerSymb  base0=LSB of Input  dbl_ovrd=off  block_type=slice
  Slice4 : xbsIndex_r4/Slice  nbits=bitPerSymb  boolean_output=off  mode=Lower Bit Location + Width  bit1=0  base1=MSB of Input  bit0=10*bitPerSymb  base0=LSB of Input  dbl_ovrd=off  block_type=slice
  Slice5 : xbsIndex_r4/Slice  nbits=bitPerSymb  boolean_output=off  mode=Lower Bit Location + Width  bit1=0  base1=MSB of Input  bit0=11*bitPerSymb  base0=LSB of Input  dbl_ovrd=off  block_type=slice
  Slice6 : xbsIndex_r4/Slice  nbits=bitPerSymb  boolean_output=off  mode=Lower Bit Location + Width  bit1=0  base1=MSB of Input  bit0=12*bitPerSymb  base0=LSB of Input  dbl_ovrd=off  block_type=slice
  Slice7 : xbsIndex_r4/Slice  nbits=bitPerSymb  boolean_output=off  mode=Lower Bit Location + Width  bit1=0  base1=MSB of Input  bit0=13*bitPerSymb  base0=LSB of Input  dbl_ovrd=off  block_type=slice
  Slice8 : xbsIndex_r4/Slice  nbits=bitPerSymb  boolean_output=off  mode=Lower Bit Location + Width  bit1=0  base1=MSB of Input  bit0=1*bitPerSymb  base0=LSB of Input  dbl_ovrd=off  block_type=slice
  Slice9 : xbsIndex_r4/Slice  nbits=bitPerSymb  boolean_output=off  mode=Lower Bit Location + Width  bit1=0  base1=MSB of Input  bit0=0*bitPerSymb  base0=LSB of Input  dbl_ovrd=off  block_type=slice
  Sub1 : Outport
  Sub2 : Outport  Port=2
  Sub3 : Outport  Port=3
  Sub4 : Outport  Port=4
  Sub5 : Outport  Port=5
  Sub6 : Outport  Port=6
  Sub7 : Outport  Port=7
  Sub8 : Outport  Port=8
  Sub9 : Outport  Port=9
  Sub10 : Outport  Port=10
  Sub11 : Outport  Port=11
  Sub12 : Outport  Port=12
  Sub13 : Outport  Port=13
  Sub14 : Outport  Port=14
  wires:
  Gateway In1/1 -> Serial to Parallel/1
  Inp/1 -> Gateway In1/1
  Slice7/1 -> Sub1/1
  Slice6/1 -> Sub2/1
  Slice5/1 -> Sub3/1
  Slice4/1 -> Sub4/1
  Slice3/1 -> Sub5/1
  Slice2/1 -> Sub6/1
  Slice1/1 -> Sub7/1
  Slice13/1 -> Sub8/1
  Slice14/1 -> Sub9/1
  Slice12/1 -> Sub10/1
  Slice11/1 -> Sub11/1
  Slice10/1 -> Sub12/1
  Slice8/1 -> Sub13/1
  Slice9/1 -> Sub14/1
  Serial to Parallel/1 -> Slice9/1, Slice8/1, Slice10/1, Slice11/1, Slice12/1, Slice14/1, Slice13/1, Slice1/1, Slice2/1, Slice3/1, Slice4/1, Slice5/1, Slice6/1, Slice7/1
